simulink model "Heli_Server"  (Simulink 7.6)
settings: Solver=ode4  SolverMode=SingleTasking  StartTime=0.0  StopTime=inf  FixedStep=0.001  MaxStep=1e-2  RelTol=1e-3
values from neighbouring files (symbols this model uses):
  D = 0.9    [exp_doc.mat]
undefined symbols (not defined in the file or in its folder): A_dlon_nom, a_mr, a_tr, B_dlat_nom, C_D0_mr, C_D0_tr, C_La_ht, C_La_vf, eps_vf_tr, g_f, g_i, gamma_fb, h_mr, h_tr, I_rot, I_xx, I_yy, I_zz, K_beta, K_i, K_mu, K_p, l_ht, l_tr, m, n_tr, Omega_nom, R_mr, R_tr, rho, s, S_ht, S_vf, S_x_fus, S_y_fus, S_z_fus, sigma_mr, sigma_tr, x0_mod
libraries: aerolib6dofsys x3, aerolibconvert2 x2, simulink x2, aerolibutil x1
settings Model: Creator=jordan  LastModifiedBy=jordan
settings DataIOCC: LimitDataPoints=off  SaveOutput=off  SignalLogging=off  DSMLogging=off  SaveTime=off
settings OptimizationCC: OptimizeModelRefInitCode=on  LifeSpan=Inf
settings HardwareCC: ProdIntDivRoundTo=Zero  ProdEndianess=LittleEndian  ProdHWDeviceType=Generic->32-bit x86 compatible
settings RTWCC: SystemTargetFile=ert.tlc  TemplateMakefile=RTW.MSVCBuild  Description=Create Visual C/C++ Solution File for the Real-Time Workshop Embedded Coder  ProcessScript=ert_make_rtw_hook  RTWCompilerOptimization=On
settings CodeAppCC: IgnoreCustomStorageClasses=off  MaxIdLength=95
settings ERTTargetCC: MultiwordLength=2048  GenerateSampleERTMain=on  LogVarNameModifier=none  MatFileLogging=on  SupportContinuousTime=on  SupportNonInlinedSFcns=on  ERTCustomFileTemplate=example_file_process.tlc  ConvertIfToSwitch=off

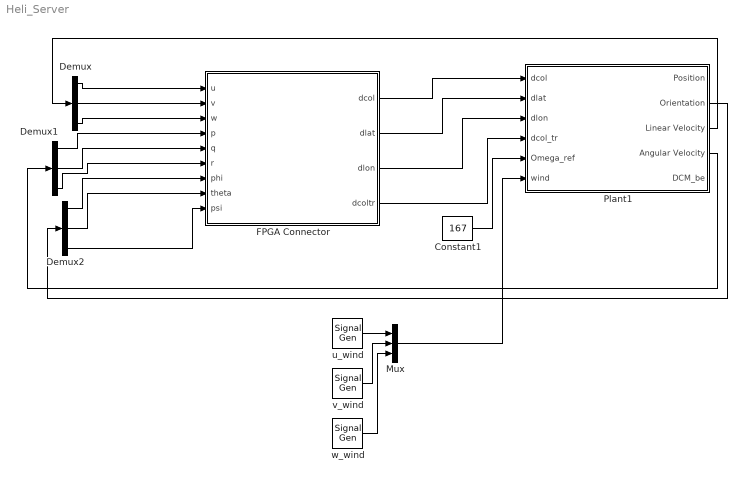
== system Heli_Server ==
  Constant1 : Constant  Value=167
  Demux : Demux  Outputs=3
  Demux1 : Demux  Outputs=3
  Demux2 : Demux  Outputs=3
  FPGA Connector : Subsystem
  Mux : Mux  Inputs=3
  Plant1 : Subsystem
  u_wind : SignalGenerator  WaveForm=square  Amplitude=5  Frequency=0.05
  v_wind : SignalGenerator  WaveForm=square  Amplitude=0.0  Frequency=0.04
  w_wind : SignalGenerator  WaveForm=square  Amplitude=0.0  Frequency=0.02
  wires:
  Plant1/3(Linear Velocity) -> Demux/1
  Plant1/4(Angular Velocity) -> Demux1/1
  Demux/1 -> FPGA Connector/1(u)
  Demux/2 -> FPGA Connector/2(v)
  Demux/3 -> FPGA Connector/3(w)
  Demux1/1 -> FPGA Connector/4(p)
  Demux1/2 -> FPGA Connector/5(q)
  Demux1/3 -> FPGA Connector/6(r)
  Demux2/1 -> FPGA Connector/7(phi)
  Demux2/2 -> FPGA Connector/8(theta)
  Demux2/3 -> FPGA Connector/9(psi)
  FPGA Connector/1(dcol) -> Plant1/1(dcol)
  FPGA Connector/4(dcoltr) -> Plant1/4(dcol_tr)
  Constant1/1 -> Plant1/5(Omega_ref)
  Plant1/2(Orientation) -> Demux2/1
  FPGA Connector/2(dlat) -> Plant1/2(dlat)
  FPGA Connector/3(dlon) -> Plant1/3(dlon)
  Mux/1 -> Plant1/6(wind)
  u_wind/1 -> Mux/1
  v_wind/1 -> Mux/2
  w_wind/1 -> Mux/3

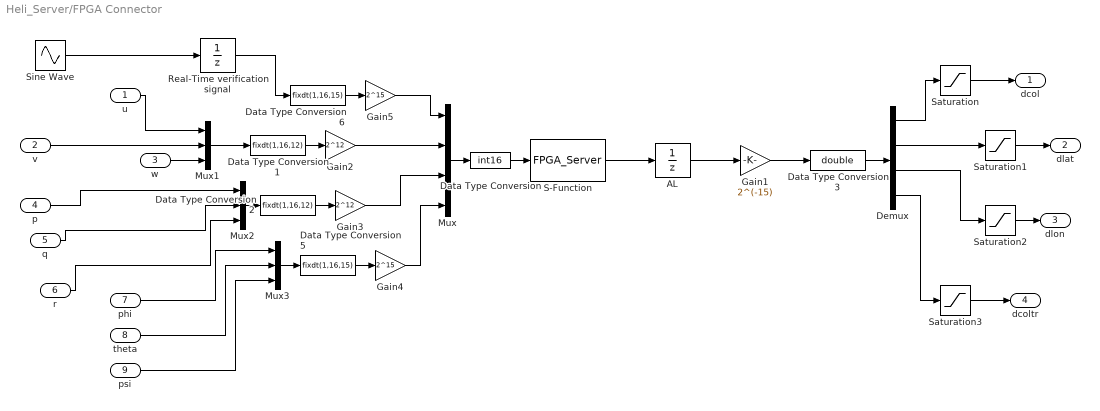
== system Heli_Server/FPGA Connector ==
  u : Inport
  v : Inport  Port=2
  w : Inport  Port=3
  p : Inport  Port=4
  q : Inport  Port=5
  r : Inport  Port=6
  phi : Inport  Port=7
  theta : Inport  Port=8
  psi : Inport  Port=9
  AL : UnitDelay  SampleTime=0.001
  Data Type Conversion : DataTypeConversion  OutDataTypeStr=int16  SaturateOnIntegerOverflow=on
  Data Type Conversion1 : DataTypeConversion  OutDataTypeStr=fixdt(1,16,12)  SaturateOnIntegerOverflow=on
  Data Type Conversion2 : DataTypeConversion  OutDataTypeStr=fixdt(1,16,12)  SaturateOnIntegerOverflow=on
  Data Type Conversion3 : DataTypeConversion  OutDataTypeStr=double  SaturateOnIntegerOverflow=on
  Data Type Conversion5 : DataTypeConversion  OutDataTypeStr=fixdt(1,16,15)  SaturateOnIntegerOverflow=on
  Data Type Conversion6 : DataTypeConversion  OutDataTypeStr=fixdt(1,16,15)  SaturateOnIntegerOverflow=on
  Demux : Demux
  Gain1 : Gain  Gain=2^(-15)  OutDataTypeStr=fixdt(1,16,15)
  Gain2 : Gain  Gain=2^12  OutDataTypeStr=int16
  Gain3 : Gain  Gain=2^12  OutDataTypeStr=int16
  Gain4 : Gain  Gain=2^15  OutDataTypeStr=int16
  Gain5 : Gain  Gain=2^15  OutDataTypeStr=int16
  Mux : Mux
  Mux1 : Mux  Inputs=3
  Mux2 : Mux  Inputs=3
  Mux3 : Mux  Inputs=3
  Real-Time verification signal : UnitDelay  SampleTime=0.001
  S-Function : S-Function  FunctionName=FPGA_Server  EnableBusSupport=off
  Saturation : Saturate  UpperLimit=0.183  LowerLimit=-0.183
  Saturation1 : Saturate  UpperLimit=0.096  LowerLimit=-0.096
  Saturation2 : Saturate  UpperLimit=0.096  LowerLimit=-0.096
  Saturation3 : Saturate  UpperLimit=0.48  LowerLimit=-0.48
  Sine Wave : Sin  Amplitude=0.3  Frequency=2*pi  SampleTime=0
  dcol : Outport
  dlat : Outport  Port=2
  dlon : Outport  Port=3
  dcoltr : Outport  Port=4
  wires:
  S-Function/1 -> AL/1
  Mux/1 -> Data Type Conversion/1
  Sine Wave/1 -> Real-Time verification signal/1
  Demux/1 -> Saturation/1
  Real-Time verification signal/1 -> Data Type Conversion6/1
  Data Type Conversion/1 -> S-Function/1
  Gain5/1 -> Mux/1
  u/1 -> Mux1/1
  v/1 -> Mux1/2
  p/1 -> Mux2/1
  q/1 -> Mux2/2
  r/1 -> Mux2/3
  phi/1 -> Mux3/1
  theta/1 -> Mux3/2
  psi/1 -> Mux3/3
  Demux/2 -> Saturation1/1
  Demux/3 -> Saturation2/1
  Demux/4 -> Saturation3/1
  Gain1/1 -> Data Type Conversion3/1
  AL/1 -> Gain1/1
  Data Type Conversion3/1 -> Demux/1
  Mux1/1 -> Data Type Conversion1/1
  Gain2/1 -> Mux/2
  Data Type Conversion2/1 -> Gain3/1
  Mux2/1 -> Data Type Conversion2/1
  Gain3/1 -> Mux/3
  Data Type Conversion5/1 -> Gain4/1
  Mux3/1 -> Data Type Conversion5/1
  Gain4/1 -> Mux/4
  Data Type Conversion6/1 -> Gain5/1
  Saturation/1 -> dcol/1
  Saturation1/1 -> dlat/1
  Saturation2/1 -> dlon/1
  Saturation3/1 -> dcoltr/1
  w/1 -> Mux1/3
  Data Type Conversion1/1 -> Gain2/1

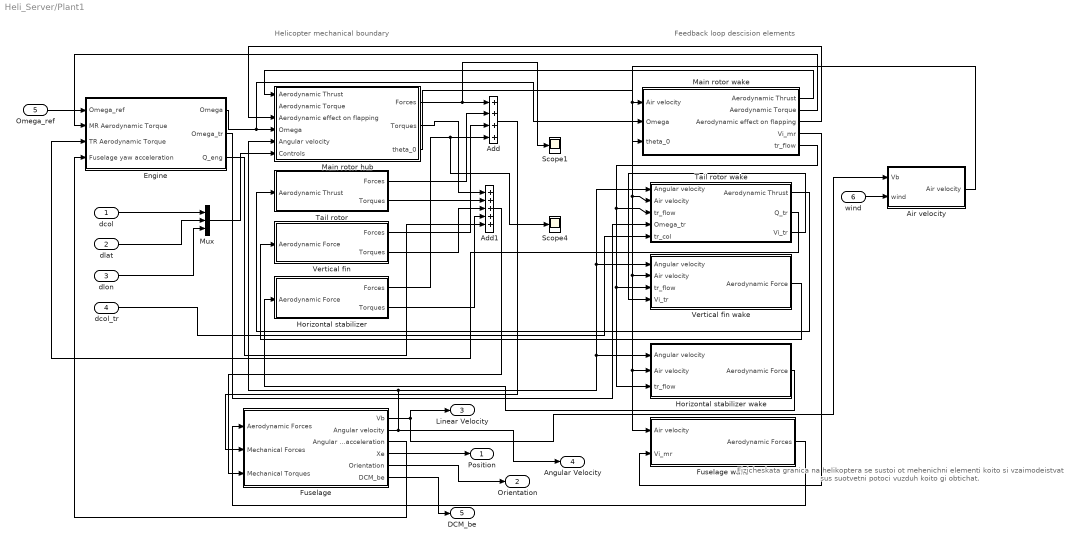
== system Heli_Server/Plant1 ==
  note: Fizicheskata granica na helikoptera
      | se sustoi ot mehenichni elementi
      | koito si vzaimodeistvat sus suotvetni
      | potoci vuzduh koito gi obtichat.
  note: Feedback loop descision elements
  note: Helicopter mechanical boundary
  dcol : Inport
  dlat : Inport  Port=2
  dlon : Inport  Port=3
  dcol_tr : Inport  Port=4
  Omega_ref : Inport  Port=5
  wind : Inport  Port=6
  Add : Sum  Inputs=++++
  Add1 : Sum  Inputs=+++++
  Air velocity : Subsystem
  Engine : Subsystem
  Fuselage : Subsystem
  Fuselage wake : Subsystem
  Horizontal stabilizer : Subsystem
  Horizontal stabilizer wake : Subsystem
  Main rotor hub : Subsystem
  Main rotor wake : Subsystem
  Mux : Mux  Inputs=3
  Scope1 : Scope
      settings: SaveName=ScopeData30
  Scope4 : Scope
      settings: SaveName=ScopeData34
  Tail rotor : Subsystem
  Tail rotor wake : Subsystem
  Vertical fin : Subsystem
  Vertical fin wake : Subsystem
  Position : Outport
  Orientation : Outport  Port=2
  Linear Velocity : Outport  Port=3
  Angular Velocity : Outport  Port=4
  DCM_be : Outport  Port=5
  wires:
  Vertical fin/1(Forces) -> Add/3
  Engine/3(Q_eng) -> Add1/5
  Tail rotor wake/2(Q_tr) -> Engine/3(TR Aerodynamic Torque)
  Fuselage/6(DCM_be) -> DCM_be/1
  wind/1 -> Air velocity/2(wind)
  Omega_ref/1 -> Engine/1(Omega_ref)
  Fuselage/5(Orientation) -> Orientation/1
  Fuselage/4(Xe) -> Position/1
  dcol_tr/1 -> Tail rotor wake/5(tr_col)
  dlon/1 -> Mux/3
  dlat/1 -> Mux/2
  dcol/1 -> Mux/1
  Horizontal stabilizer/2(Torques) -> Add1/4
  Vertical fin/2(Torques) -> Add1/3
  Tail rotor/2(Torques) -> Add1/2
  Main rotor hub/2(Torques) -> Add1/1
  Add1/1 -> Fuselage/3(Mechanical Torques)
  Horizontal stabilizer/1(Forces) -> Scope4/1, Add/4
  Tail rotor/1(Forces) -> Add/2
  Add/1 -> Fuselage/2(Mechanical Forces)
  Horizontal stabilizer wake/1(Aerodynamic Force) -> Horizontal stabilizer/1(Aerodynamic Force)
  Vertical fin wake/1(Aerodynamic Force) -> Vertical fin/1(Aerodynamic Force)
  Tail rotor wake/1(Aerodynamic Thrust) -> Tail rotor/1(Aerodynamic Thrust)
  Engine/2(Omega_tr) -> Tail rotor wake/4(Omega_tr)
  Main rotor wake/5(tr_flow) -> Tail rotor wake/3(tr_flow), Horizontal stabilizer wake/3(tr_flow), Vertical fin wake/3(tr_flow)
  Mux/1 -> Main rotor hub/6(Controls)
  Main rotor hub/1(Forces) -> Scope1/1, Add/1
  Main rotor hub/3(theta_0) -> Main rotor wake/3(theta_0)
  Main rotor wake/3(Aerodynamic effect on flapping) -> Main rotor hub/3(Aerodynamic effect on flapping)
  Fuselage/3(Angular acceleration) -> Engine/4(Fuselage yaw acceleration)
  Tail rotor wake/3(Vi_tr) -> Vertical fin wake/4(Vi_tr)
  Fuselage/2(Angular velocity) -> Angular Velocity/1, Horizontal stabilizer wake/1(Angular velocity), Tail rotor wake/1(Angular velocity), Vertical fin wake/1(Angular velocity), Main rotor hub/5(Angular velocity)
  Fuselage wake/1(Aerodynamic Forces) -> Fuselage/1(Aerodynamic Forces)
  Main rotor wake/4(Vi_mr) -> Fuselage wake/2(Vi_mr)
  Main rotor wake/2(Aerodynamic Torque) -> Engine/2(MR Aerodynamic Torque)
  Air velocity/1(Air velocity) -> Main rotor wake/1(Air velocity), Tail rotor wake/2(Air velocity), Horizontal stabilizer wake/2(Air velocity), Fuselage wake/1(Air velocity), Vertical fin wake/2(Air velocity)
  Fuselage/1(Vb) -> Linear Velocity/1, Air velocity/1(Vb)
  Main rotor wake/1(Aerodynamic Thrust) -> Main rotor hub/1(Aerodynamic Thrust)
  Engine/1(Omega) -> Main rotor wake/2(Omega), Main rotor hub/4(Omega)

== system Heli_Server/Plant1/Air velocity ==
  Vb : Inport
  wind : Inport  Port=2
  Add : Sum  Inputs=-+
  Air velocity : Outport
  wires:
  Add/1 -> Air velocity/1
  Vb/1 -> Add/2
  wind/1 -> Add/1

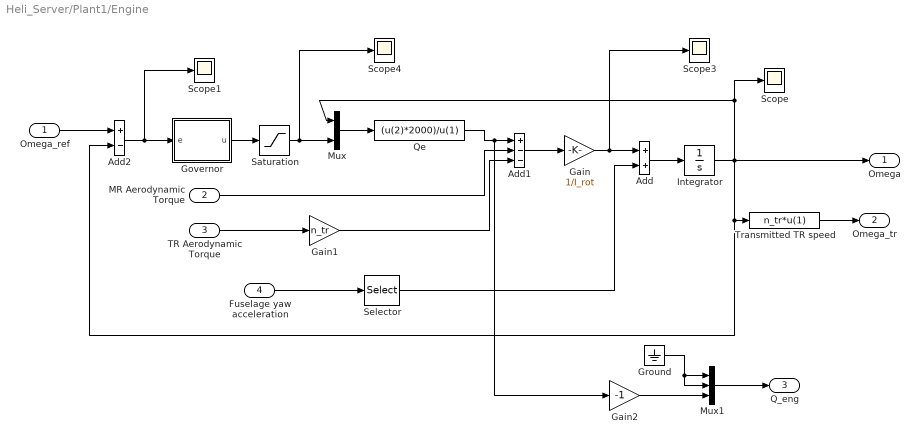
== system Heli_Server/Plant1/Engine ==
  Omega_ref : Inport
  MR Aerodynamic Torque : Inport  Port=2
  TR Aerodynamic Torque : Inport  Port=3
  Fuselage yaw acceleration : Inport  Port=4
  Add : Sum
  Add1 : Sum  Inputs=+--
  Add2 : Sum  Inputs=+-
  Gain : Gain  Gain=1/I_rot
  Gain1 : Gain  Gain=n_tr
  Gain2 : Gain  Gain=-1
  Governor : Subsystem
  Ground : Ground
  Integrator : Integrator  InitialCondition=167  UpperSaturationLimit=200  LowerSaturationLimit=150  ContinuousStateAttributes='Omega'
  Mux : Mux  Inputs=2
  Mux1 : Mux  Inputs=3
  Qe : Fcn  Expr=(u(2)*2000)/u(1)
  Saturation : Saturate  UpperLimit=1  LowerLimit=-1
  Scope{,1,3..4} (4 alike) : Scope
      Scope settings: TimeRange=10  YMin=166  YMax=168.5  SaveName=ScopeData28
      Scope1 settings: TimeRange=10  YMin=-1.5  YMax=0.25  SaveName=ScopeData31
      Scope3 settings: TimeRange=10  YMin=166  YMax=168.5  SaveName=ScopeData26
      Scope4 settings: TimeRange=10  YMin=-1.5  YMax=0.25  SaveName=ScopeData27
  Selector : Selector  InputPortWidth=3  IndexOptions=Index vector (dialog)  Indices=3  OutputSizes=1
  Transmitted TR speed : Fcn  Expr=n_tr*u(1)
  Omega : Outport
  Omega_tr : Outport  Port=2
  Q_eng : Outport  Port=3
  wires:
  Mux1/1 -> Q_eng/1
  Ground/1 -> Mux1/2, Mux1/1
  Gain2/1 -> Mux1/3
  Gain1/1 -> Add1/3
  Mux/1 -> Qe/1
  Qe/1 -> Gain2/1, Add1/1
  Saturation/1 -> Scope4/1, Mux/2
  Governor/1(u) -> Saturation/1
  Add2/1 -> Governor/1(e), Scope1/1
  Omega_ref/1 -> Add2/1
  TR Aerodynamic Torque/1 -> Gain1/1
  MR Aerodynamic Torque/1 -> Add1/2
  Gain/1 -> Scope3/1, Add/1
  Add1/1 -> Gain/1
  Selector/1 -> Add/2
  Add/1 -> Integrator/1
  Fuselage yaw acceleration/1 -> Selector/1
  Transmitted TR speed/1 -> Omega_tr/1
  Integrator/1 -> Omega/1, Mux/1, Scope/1, Add2/2, Transmitted TR speed/1

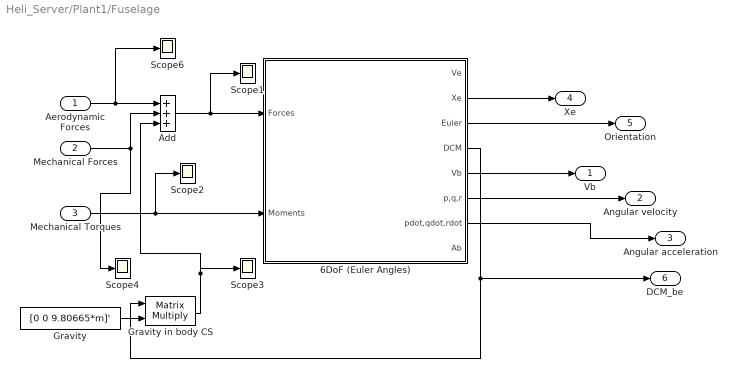
== system Heli_Server/Plant1/Fuselage ==
  Aerodynamic Forces : Inport
  Mechanical Forces : Inport  Port=2
  Mechanical Torques : Inport  Port=3
  6DoF (Euler Angles) : Subsystem  AncestorBlock=aerolib6dof2/6DoF (Euler Angles)  mask(6DoF EoM (Body Axis)){units=Metric (MKS), mtype=Fixed, rep=Euler Angles, xme_0=[0 0 0], Vm_0=[0 0 0], eul_0=[0 0 0], pm_0=[0 0 0], mass_0=m, mass_e=0.5, mass_f=2.0, inertia=[I_xx 0 0;0 I_yy 0;0 0 I_zz], inertia_e=eye(3), inertia_f=2*eye(3), k_quat=1.0}
      mask prompts: mtype "Mass type:"; rep "Representation:"; xme_0 "Initial position in inertial axes [Xe,Ye,Ze]:"; Vm_0 "Initial velocity in body axes [U,v,w]:"; eul_0 "Initial Euler orientation [roll, pitch, yaw]:"; pm_0 "Initial body rotation rates [p,q,r]:"; mass_0 "Initial mass:"; mass_e "Empty mass:"; mass_f "Full mass:"; inertia_e "Empty inertia matrix:"; inertia_f "Full inertia matrix:"; k_quat "Gain for quaternion normalization:"
      mask help: Integrate the six-degrees-of-freedom equations of motion in body axis.
      mask init:
      | [x y xp yp highstr lowstr maxy miny]=aeroimage('sixdofbody',gcbh);
      | ports=aeroicon('aeroblk6dofbody','icon');
      mask Help: eval('asbhelp(''sixdof_euler_angles'')');
      mask StyleString: popup(Metric (MKS)|English (Velocity in ft/s)|English (Velocity in kts)),popup(Fixed|Simple Variable|Custom Variable),popup(Euler Angles|Quaternion),edit,edit,edit,edit,edit,edit,edit,edit,edit,edit,edit
      mask CallbackString: |aeroicon('aeroblk6dofbody');|aeroicon('aeroblk6dofbody');|||||||||||
      mask Display:
      | port_label(ports(1).type,ports(1).port,ports(1).txt,'texmode','on');
      | port_label(ports(2).type,ports(2).port,ports(2).txt,'texmode','on');
      | port_label(ports(3).type,ports(3).port,ports(3).txt,'texmode','on');
      | port_label(ports(4).type,ports(4).port,ports(4).txt,'texmode','on');
      | port_label(ports(5).type,ports(5).port,ports(5).txt,'texmode','on');
      | port_label(ports(6).type,ports(6).port,ports(6).txt,'texmode','on');
      | port_label(ports(7).type,ports(7).port,ports(7).txt,'texmode','on');
      | port_label(ports(8).type,ports(8).port,ports(8).txt,'texmode','on');
      | port_label(ports(9).type,ports(9).port,ports(9).txt,'texmode','on');
      | port_label(ports(10).type,ports(10).port,ports(10).txt,'texmode','on');
      | port_label(ports(11).type,ports(11).port,ports(11).txt,'texmode','on');
      | port_label(ports(12).type,ports(12).port,ports(12).txt,'texmode','on');
      | port_label(ports(13).type,ports(13).port,ports(13).txt,'texmode','on');
      | port_label(ports(14).type,ports(14).port,ports(14).txt,'texmode','on');
      | port_label(ports(15).type,ports(15).port,ports(15).txt,'texmode','on');
      | text(0.5,maxy+0.065,highstr{:},'horizontalAlignment','center')
      | text(0.5,miny-0.05,lowstr{:},'horizontalAlignment','center')
      | plot(x,y);
      | patch(xp, yp);
  Add : Sum  Inputs=+++
  Gravity : Constant  Value=[0 0 9.80665*m]'
  Gravity in body CS : Product  Multiplication=Matrix(*)  RndMeth=Zero
  Scope{1..4,6} (5 alike) : Scope
      Scope3 settings: SaveName=ScopeData19
      Scope4 settings: SaveName=ScopeData29
      Scope6 settings: SaveName=ScopeData23
  Vb : Outport
  Angular velocity : Outport  Port=2
  Angular acceleration : Outport  Port=3
  Xe : Outport  Port=4
  Orientation : Outport  Port=5
  DCM_be : Outport  Port=6
  wires:
  6DoF (Euler Angles)/3(Euler) -> Orientation/1
  6DoF (Euler Angles)/2(Xe) -> Xe/1
  Gravity in body CS/1 -> Scope3/1, Add/3
  Gravity/1 -> Gravity in body CS/2
  6DoF (Euler Angles)/4(DCM) -> DCM_be/1, Gravity in body CS/1
  6DoF (Euler Angles)/5(Vb) -> Vb/1
  6DoF (Euler Angles)/7(pdot,qdot,rdot) -> Angular acceleration/1
  6DoF (Euler Angles)/6(p,q,r) -> Angular velocity/1
  Mechanical Torques/1 -> 6DoF (Euler Angles)/2(Moments), Scope2/1
  Add/1 -> 6DoF (Euler Angles)/1(Forces), Scope1/1
  Mechanical Forces/1 -> Scope4/1, Add/2
  Aerodynamic Forces/1 -> Add/1, Scope6/1

== system Heli_Server/Plant1/Fuselage wake ==
  Air velocity : Inport
  Vi_mr : Inport  Port=2
  Mux : Mux  Inputs=2
  Mux1 : Mux  Inputs=3
  Mux2 : Mux  Inputs=2
  V_inf : Fcn  Expr=sqrt(u(1)^2+u(2)^2+(u(3)+u(4))^2)
  X_fus : Fcn  Expr=-0.5*rho*S_x_fus*u(1)*u(5)
  Y_fus : Fcn  Expr=-0.5*rho*S_y_fus*u(2)*u(5)
  Z_fus : Fcn  Expr=-0.5*rho*S_z_fus*(u(3)+u(4))*u(5)
  Aerodynamic Forces : Outport
  wires:
  Z_fus/1 -> Mux1/3
  Y_fus/1 -> Mux1/2
  X_fus/1 -> Mux1/1
  Mux2/1 -> Z_fus/1, Y_fus/1, X_fus/1
  V_inf/1 -> Mux2/2
  Mux1/1 -> Aerodynamic Forces/1
  Mux/1 -> Mux2/1, V_inf/1
  Vi_mr/1 -> Mux/2
  Air velocity/1 -> Mux/1

== system Heli_Server/Plant1/Horizontal stabilizer ==
  Aerodynamic Force : Inport
  Ground : Ground
  Mux : Mux  Inputs=3
  Mux1 : Mux  Inputs=3
  pitch torque : Fcn  Expr=u(1)*l_ht
  Forces : Outport
  Torques : Outport  Port=2
  wires:
  pitch torque/1 -> Mux1/2
  Mux/1 -> Forces/1
  Aerodynamic Force/1 -> Mux/3, pitch torque/1
  Ground/1 -> Mux/2, Mux1/1, Mux1/3, Mux/1
  Mux1/1 -> Torques/1

== system Heli_Server/Plant1/Horizontal stabilizer wake ==
  Angular velocity : Inport
  Air velocity : Inport  Port=2
  tr_flow : Inport  Port=3
  Gain : Gain  Gain=-1
  Mux : Mux  Inputs=3
  Mux2 : Mux  Inputs=2
  Z_ht : simulink/Discontinuities/Saturation Dynamic  SystemSampleTime=-1  OutMin=[]  OutMax=[]  OutDataTypeStr=Inherit: Same as second input  OutDataType=fixdt(1, 16)  OutScaling=2^-10  DoSatur=off
  Z_ht_ideal : Fcn  Expr=0.5*rho*S_ht*(C_La_ht*abs(u(1))*u(4)+abs(u(4))*u(4))
  Z_ht_max : Fcn  Expr=0.5*rho*S_ht*(u(1)^2+u(4)^2)
  w_ht : Fcn  Expr=u(6)+l_ht*u(2)-u(7)
  Aerodynamic Force : Outport
  wires:
  Z_ht/1 -> Aerodynamic Force/1
  Gain/1 -> Z_ht/3
  Z_ht_max/1 -> Gain/1, Z_ht/1
  Z_ht_ideal/1 -> Z_ht/2
  Mux2/1 -> Z_ht_max/1, Z_ht_ideal/1
  w_ht/1 -> Mux2/2
  tr_flow/1 -> Mux/3
  Air velocity/1 -> Mux2/1, Mux/2
  Angular velocity/1 -> Mux/1
  Mux/1 -> w_ht/1

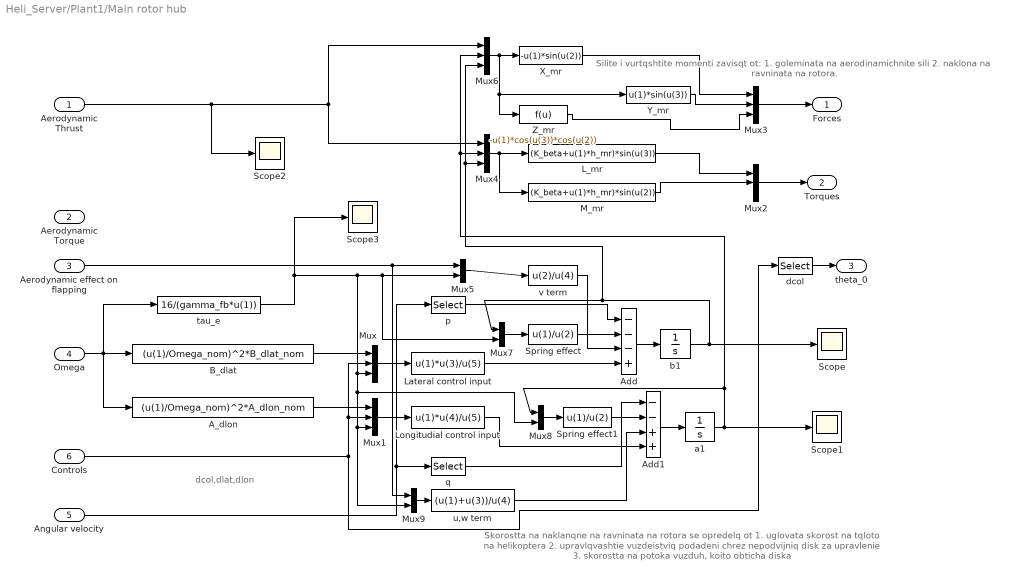
== system Heli_Server/Plant1/Main rotor hub ==
  note: dcol,dlat,dlon
  note: Skorostta na naklanqne na ravninata na rotora se opredelq ot
      | 1. uglovata skorost na tqloto na helikoptera
      | 2. upravlqvashtie vuzdeistviq podadeni chrez
      | nepodvijniq disk za upravlenie
      | 3. skorostta na potoka vuzduh, koito obticha diska
  note: Silite i vurtqshtite momenti zavisqt ot:
      | 1. goleminata na aerodinamichnite sili
      | 2. naklona na ravninata na rotora.
  Aerodynamic Thrust : Inport
  Aerodynamic Torque : Inport  Port=2
  Aerodynamic effect on flapping : Inport  Port=3
  Omega : Inport  Port=4
  Angular velocity : Inport  Port=5
  Controls : Inport  Port=6
  A_dlon : Fcn  Expr=(u(1)/Omega_nom)^2*A_dlon_nom
  Add : Sum  Inputs=---+
  Add1 : Sum  Inputs=--++
  B_dlat : Fcn  Expr=(u(1)/Omega_nom)^2*B_dlat_nom
  L_mr : Fcn  Expr=(K_beta+u(1)*h_mr)*sin(u(3))
  Lateral control input : Fcn  Expr=u(1)*u(3)/u(5)
  Longitudial control input : Fcn  Expr=u(1)*u(4)/u(5)
  M_mr : Fcn  Expr=(K_beta+u(1)*h_mr)*sin(u(2))
  Mux{,1..4,6} (6 alike) : Mux  Inputs=3
  Mux{5,7..9} (4 alike) : Mux  Inputs=2
  Scope{,1..3} (4 alike) : Scope
      Scope settings: SaveName=ScopeData2
      Scope1 settings: SaveName=ScopeData3
      Scope2 settings: SaveName=ScopeData35
      Scope3 settings: SaveName=ScopeData18
  Spring effect : Fcn  Expr=u(1)/u(2)
  Spring effect1 : Fcn  Expr=u(1)/u(2)
  X_mr : Fcn  Expr=-u(1)*sin(u(2))
  Y_mr : Fcn  Expr=u(1)*sin(u(3))
  Z_mr : Fcn  Expr=-u(1)*cos(u(3))*cos(u(2))
  a1 : Integrator  InitialCondition=x0_mod(12)
  b1 : Integrator  InitialCondition=x0_mod(13)
  dcol : Selector  InputPortWidth=3  IndexOptions=Index vector (dialog)  Indices=1  OutputSizes=1
  p : Selector  InputPortWidth=3  IndexOptions=Index vector (dialog)  Indices=1  OutputSizes=1
  q : Selector  InputPortWidth=3  IndexOptions=Index vector (dialog)  Indices=2  OutputSizes=1
  tau_e : Fcn  Expr=16/(gamma_fb*u(1))
  u,w term : Fcn  Expr=(u(1)+u(3))/u(4)
  v term : Fcn  Expr=u(2)/u(4)
  Forces : Outport
  Torques : Outport  Port=2
  theta_0 : Outport  Port=3
  wires:
  Mux9/1 -> u,w term/1
  Mux8/1 -> Spring effect1/1
  Mux7/1 -> Spring effect/1
  tau_e/1 -> Scope3/1, Mux9/2, Mux1/3, Mux8/2, Mux/3, Mux7/2, Mux5/2
  Mux5/1 -> v term/1
  Aerodynamic effect on flapping/1 -> Mux9/1, Mux5/1
  dcol/1 -> theta_0/1
  Z_mr/1 -> Mux3/3
  Y_mr/1 -> Mux3/2
  X_mr/1 -> Mux3/1
  Mux6/1 -> Z_mr/1, Y_mr/1, X_mr/1
  M_mr/1 -> Mux2/2
  L_mr/1 -> Mux2/1
  Aerodynamic Thrust/1 -> Scope2/1, Mux6/1, Mux4/1
  Mux4/1 -> M_mr/1, L_mr/1
  Mux3/1 -> Forces/1
  Mux2/1 -> Torques/1
  Longitudial control input/1 -> Add1/4
  Spring effect1/1 -> Add1/2
  Add1/1 -> a1/1
  u,w term/1 -> Add1/3
  a1/1 -> Scope1/1, Mux8/1, Mux4/2, Mux6/2
  q/1 -> Add1/1
  Angular velocity/1 -> q/1, p/1
  v term/1 -> Add/3
  Spring effect/1 -> Add/2
  b1/1 -> Scope/1, Mux7/1, Mux4/3, Mux6/3
  Add/1 -> b1/1
  Lateral control input/1 -> Add/4
  p/1 -> Add/1
  Mux1/1 -> Longitudial control input/1
  A_dlon/1 -> Mux1/1
  Mux/1 -> Lateral control input/1
  Controls/1 -> dcol/1, Mux/2, Mux1/2
  B_dlat/1 -> Mux/1
  Omega/1 -> tau_e/1, A_dlon/1, B_dlat/1

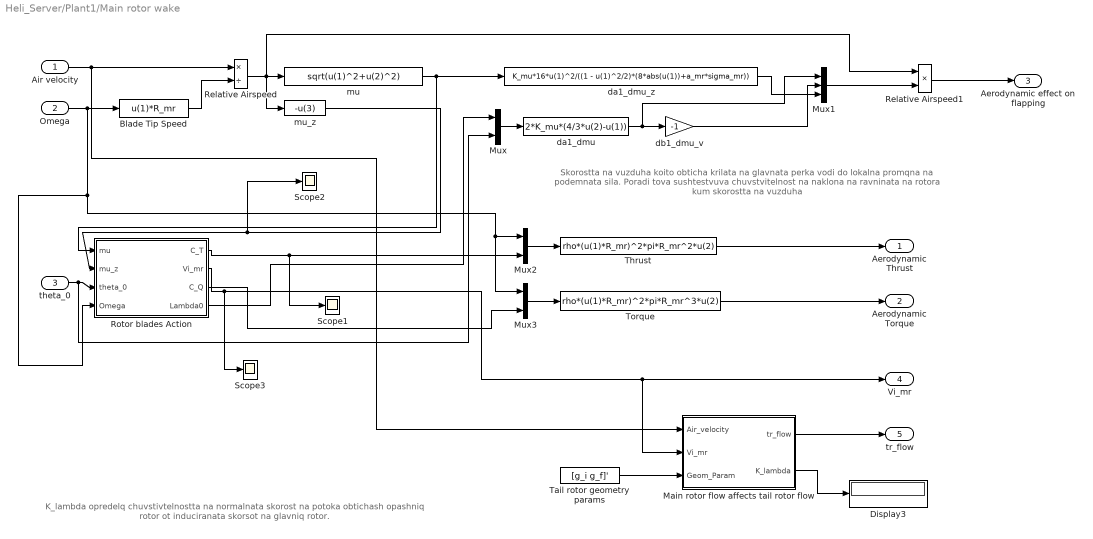
== system Heli_Server/Plant1/Main rotor wake ==
  note: Skorostta na vuzduha koito obticha krilata na glavnata
      | perka vodi do lokalna promqna na podemnata sila.
      | Poradi tova sushtestvuva chuvstvitelnost na naklona
      | na ravninata na rotora kum skorostta na vuzduha
  note: K_lambda opredelq chuvstivtelnostta na
      | normalnata skorost na potoka obtichash
      | opashniq rotor ot induciranata skorsot na
      | glavniq rotor.
  Air velocity : Inport  PortDimensions=3
  Omega : Inport  Port=2
  theta_0 : Inport  Port=3
  Blade Tip Speed : Fcn  Expr=u(1)*R_mr
  Display3 : Display
  Main rotor flow affects tail rotor flow : Stateflow chart  TreatAsAtomicUnit=on
  Mux : Mux  Inputs=2
  Mux1 : Mux  Inputs=3
  Mux2 : Mux  Inputs=2
  Mux3 : Mux  Inputs=2
  Relative Airspeed : Product  Inputs=*/
  Relative Airspeed1 : Product  Inputs=**
  Rotor blades Action : Subsystem
  Scope1 : Scope
      settings: SaveName=ScopeData11
  Scope2 : Scope
      settings: SaveName=ScopeData10
  Scope3 : Scope
      settings: SaveName=ScopeData12
  Tail rotor geometry params : Constant  Value=[g_i g_f]'
  Thrust : Fcn  Expr=rho*(u(1)*R_mr)^2*pi*R_mr^2*u(2)
  Torque : Fcn  Expr=rho*(u(1)*R_mr)^2*pi*R_mr^3*u(2)
  da1_dmu : Fcn  Expr=2*K_mu*(4/3*u(2)-u(1))
  da1_dmu_z : Fcn  Expr=K_mu*16*u(1)^2/((1 - u(1)^2/2)*(8*abs(u(1))+a_mr*sigma_mr))
  db1_dmu_v : Gain  Gain=-1
  mu : Fcn  Expr=sqrt(u(1)^2+u(2)^2)
  mu_z : Fcn  Expr=-u(3)
  Aerodynamic Thrust : Outport
  Aerodynamic Torque : Outport  Port=2
  Aerodynamic effect on flapping : Outport  Port=3
  Vi_mr : Outport  Port=4
  tr_flow : Outport  Port=5
  wires:
  Main rotor flow affects tail rotor flow/2(K_lambda) -> Display3/1
  Mux3/1 -> Torque/1
  Torque/1 -> Aerodynamic Torque/1
  Air velocity/1 -> Relative Airspeed/1, Main rotor flow affects tail rotor flow/1(Air_velocity)
  Omega/1 -> Rotor blades Action/4(Omega), Mux3/1, Mux2/1, Blade Tip Speed/1
  Blade Tip Speed/1 -> Relative Airspeed/2
  Relative Airspeed/1 -> mu/1, mu_z/1, Relative Airspeed1/1
  mu/1 -> Rotor blades Action/1(mu), da1_dmu_z/1
  mu_z/1 -> Rotor blades Action/2(mu_z), Scope2/1
  theta_0/1 -> Rotor blades Action/3(theta_0), Mux/2
  Mux/1 -> da1_dmu/1
  Rotor blades Action/2(Vi_mr) -> Scope3/1, Vi_mr/1, Main rotor flow affects tail rotor flow/2(Vi_mr)
  da1_dmu/1 -> db1_dmu_v/1, Mux1/1
  da1_dmu_z/1 -> Mux1/3
  db1_dmu_v/1 -> Mux1/2
  Rotor blades Action/1(C_T) -> Mux2/2, Scope1/1
  Mux2/1 -> Thrust/1
  Thrust/1 -> Aerodynamic Thrust/1
  Rotor blades Action/3(C_Q) -> Mux3/2
  Main rotor flow affects tail rotor flow/1(tr_flow) -> tr_flow/1
  Tail rotor geometry params/1 -> Main rotor flow affects tail rotor flow/3(Geom_Param)
  Rotor blades Action/4(Lambda0) -> Mux/1
  Relative Airspeed1/1 -> Aerodynamic effect on flapping/1
  Mux1/1 -> Relative Airspeed1/2

== system Heli_Server/Plant1/Tail rotor ==
  note: Vurhu opashniqt rotor deistva tqgata
      | poluchena ot vurteneto na perkata.
      | Tova suzdava mehanichni sili vurhu tqloto
      | na helikoptera.
  Aerodynamic Thrust : Inport
  Ground : Ground
  Mux : Mux  Inputs=3
  Mux1 : Mux  Inputs=3
  roll torque : Fcn  Expr=u(1)*h_tr
  yaw torque : Fcn  Expr=-u(1)*l_tr
  Forces : Outport
  Torques : Outport  Port=2
  wires:
  roll torque/1 -> Mux1/1
  yaw torque/1 -> Mux1/3
  Mux1/1 -> Torques/1
  Ground/1 -> Mux1/2, Mux/3, Mux/1
  Aerodynamic Thrust/1 -> roll torque/1, yaw torque/1, Mux/2
  Mux/1 -> Forces/1

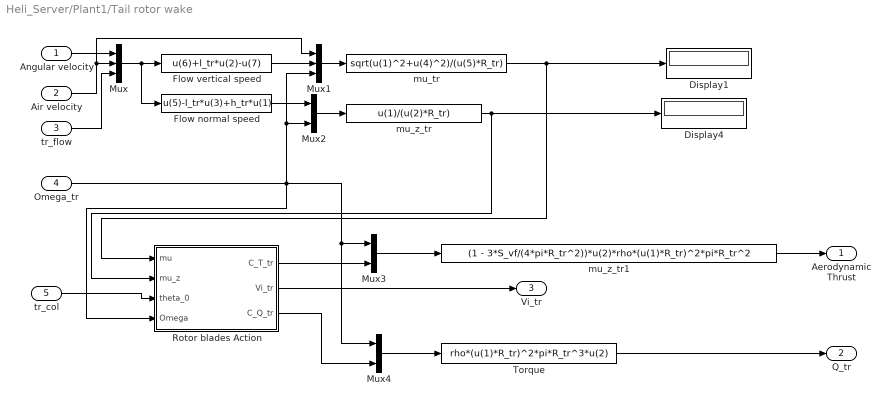
== system Heli_Server/Plant1/Tail rotor wake ==
  Angular velocity : Inport
  Air velocity : Inport  Port=2
  tr_flow : Inport  Port=3
  Omega_tr : Inport  Port=4
  tr_col : Inport  Port=5
  Display1 : Display
  Display4 : Display
  Flow normal speed : Fcn  Expr=u(5)-l_tr*u(3)+h_tr*u(1)
  Flow vertical speed : Fcn  Expr=u(6)+l_tr*u(2)-u(7)
  Mux : Mux  Inputs=3
  Mux1 : Mux  Inputs=3
  Mux2 : Mux  Inputs=2
  Mux3 : Mux  Inputs=2
  Mux4 : Mux  Inputs=2
  Rotor blades Action : Subsystem
  Torque : Fcn  Expr=rho*(u(1)*R_tr)^2*pi*R_tr^3*u(2)
  mu_tr : Fcn  Expr=sqrt(u(1)^2+u(4)^2)/(u(5)*R_tr)
  mu_z_tr : Fcn  Expr=u(1)/(u(2)*R_tr)
  mu_z_tr1 : Fcn  Expr=(1 - 3*S_vf/(4*pi*R_tr^2))*u(2)*rho*(u(1)*R_tr)^2*pi*R_tr^2
  Aerodynamic Thrust : Outport
  Q_tr : Outport  Port=2
  Vi_tr : Outport  Port=3
  wires:
  Air velocity/1 -> Mux/2, Mux1/1
  Angular velocity/1 -> Mux/1
  tr_flow/1 -> Mux/3
  Mux/1 -> Flow normal speed/1, Flow vertical speed/1
  Omega_tr/1 -> Rotor blades Action/4(Omega), Mux3/1, Mux4/1, Mux1/3, Mux2/2
  Mux1/1 -> mu_tr/1
  Mux2/1 -> mu_z_tr/1
  tr_col/1 -> Rotor blades Action/3(theta_0)
  mu_z_tr/1 -> Rotor blades Action/2(mu_z), Display4/1
  mu_z_tr1/1 -> Aerodynamic Thrust/1
  mu_tr/1 -> Rotor blades Action/1(mu), Display1/1
  Rotor blades Action/2(Vi_tr) -> Vi_tr/1
  Rotor blades Action/1(C_T_tr) -> Mux3/2
  Mux3/1 -> mu_z_tr1/1
  Torque/1 -> Q_tr/1
  Mux4/1 -> Torque/1
  Rotor blades Action/3(C_Q_tr) -> Mux4/2
  Flow vertical speed/1 -> Mux1/2
  Flow normal speed/1 -> Mux2/1

== system Heli_Server/Plant1/Vertical fin ==
  Aerodynamic Force : Inport
  Ground : Ground
  Mux : Mux  Inputs=3
  Mux1 : Mux  Inputs=3
  roll torque : Fcn  Expr=u(1)*h_tr
  yaw torque : Fcn  Expr=-u(1)*l_tr
  Forces : Outport
  Torques : Outport  Port=2
  wires:
  roll torque/1 -> Mux1/1
  yaw torque/1 -> Mux1/3
  Mux1/1 -> Torques/1
  Ground/1 -> Mux1/2, Mux/3, Mux/1
  Aerodynamic Force/1 -> roll torque/1, yaw torque/1, Mux/2
  Mux/1 -> Forces/1

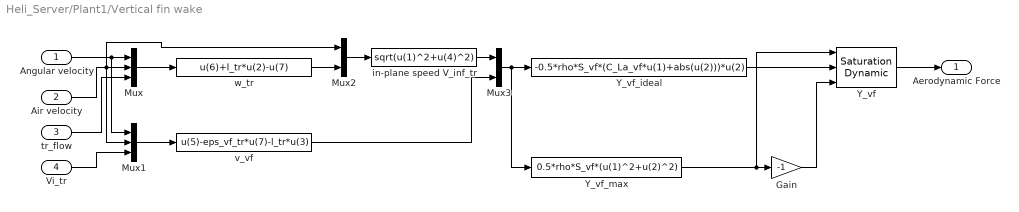
== system Heli_Server/Plant1/Vertical fin wake ==
  Angular velocity : Inport
  Air velocity : Inport  Port=2
  tr_flow : Inport  Port=3
  Vi_tr : Inport  Port=4
  Gain : Gain  Gain=-1
  Mux : Mux  Inputs=3
  Mux1 : Mux  Inputs=3
  Mux2 : Mux  Inputs=2
  Mux3 : Mux  Inputs=2
  Y_vf : simulink/Discontinuities/Saturation Dynamic  SystemSampleTime=-1  OutMin=[]  OutMax=[]  OutDataTypeStr=Inherit: Same as second input  OutDataType=fixdt(1, 16)  OutScaling=2^-10  DoSatur=off
  Y_vf_ideal : Fcn  Expr=-0.5*rho*S_vf*(C_La_vf*u(1)+abs(u(2)))*u(2)
  Y_vf_max : Fcn  Expr=0.5*rho*S_vf*(u(1)^2+u(2)^2)
  in-plane speed V_inf_tr : Fcn  Expr=sqrt(u(1)^2+u(4)^2)
  v_vf : Fcn  Expr=u(5)-eps_vf_tr*u(7)-l_tr*u(3)
  w_tr : Fcn  Expr=u(6)+l_tr*u(2)-u(7)
  Aerodynamic Force : Outport
  wires:
  Y_vf/1 -> Aerodynamic Force/1
  Gain/1 -> Y_vf/3
  Y_vf_max/1 -> Gain/1, Y_vf/1
  Y_vf_ideal/1 -> Y_vf/2
  Mux3/1 -> Y_vf_max/1, Y_vf_ideal/1
  v_vf/1 -> Mux3/2
  in-plane speed V_inf_tr/1 -> Mux3/1
  Mux2/1 -> in-plane speed V_inf_tr/1
  w_tr/1 -> Mux2/2
  Mux1/1 -> v_vf/1
  Vi_tr/1 -> Mux1/3
  tr_flow/1 -> Mux/3
  Air velocity/1 -> Mux2/1, Mux1/2, Mux/2
  Angular velocity/1 -> Mux1/1, Mux/1
  Mux/1 -> w_tr/1

== system Heli_Server/Plant1/Engine/Governor ==
  e : Inport
  Add3 : Sum
  Gain3 : Gain  Gain=K_p
  Gain4 : Gain  Gain=K_i
  Integrator1 : Integrator  InitialCondition=x0_mod(11)  UpperSaturationLimit=200  LowerSaturationLimit=150  ContinuousStateAttributes='Omega'
  Scope1 : Scope
      settings: TimeRange=10  YMin=-1.5  YMax=0.25  SaveName=ScopeData15
  u : Outport
  wires:
  Gain4/1 -> Scope1/1, Add3/2
  Add3/1 -> u/1
  e/1 -> Integrator1/1, Gain3/1
  Integrator1/1 -> Gain4/1
  Gain3/1 -> Add3/1

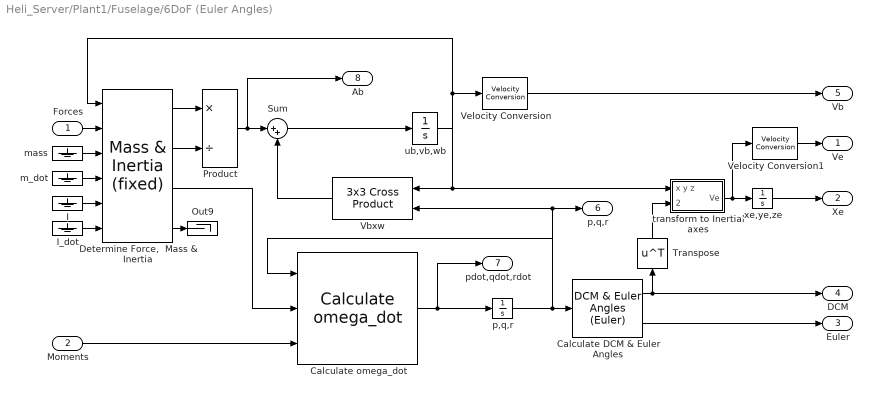
== system Heli_Server/Plant1/Fuselage/6DoF (Euler Angles) ==
  Forces : Inport
  Moments : Inport  Port=2
  Calculate DCM & Euler Angles : aerolib6dofsys/DCM & Euler Angles (Euler)  SystemSampleTime=-1
  Calculate omega_dot : aerolib6dofsys/Calculate omega_dot  SystemSampleTime=-1
  "Determine Force,  Mass & Inertia" : aerolib6dofsys/Mass & Inertia (fixed)  SystemSampleTime=-1
  I : Ground
  I_dot : Ground
  Out9 : Terminator
  Product : Product  Inputs=*/  SaturateOnIntegerOverflow=on  OutDataTypeStr=Inherit: Same as first input
  Sum : Sum  Inputs=|++  SaturateOnIntegerOverflow=on
  Transpose : Math  Operator=transpose  SaturateOnIntegerOverflow=on
  Vbxw : aerolibutil/3x3 Cross Product  SystemSampleTime=-1
  Velocity Conversion : aerolibconvert2/Velocity Conversion  SystemSampleTime=-1  IU=m/s  OU=m/s
  Velocity Conversion1 : aerolibconvert2/Velocity Conversion  SystemSampleTime=-1  IU=m/s  OU=m/s
  m_dot : Ground
  mass : Ground
  "p,q,r " : Integrator  InitialCondition=pm_0
  "transform to Inertial axes " : Subsystem
      mask Type: Vector Transformation
      mask Display: disp('L_EB')
  ub,vb,wb : Integrator  InitialCondition=convvel(Vm_0,'m/s','m/s')
  xe,ye,ze : Integrator  InitialCondition=xme_0
  Ve : Outport
  Xe : Outport  Port=2
  Euler : Outport  Port=3
  DCM : Outport  Port=4
  Vb : Outport  Port=5
  p,q,r : Outport  Port=6
  pdot,qdot,rdot : Outport  Port=7
  Ab : Outport  Port=8
  wires:
  Velocity Conversion1/1 -> Ve/1
  Velocity Conversion/1 -> Vb/1
  "Determine Force,  Mass & Inertia"/3 -> Calculate omega_dot/2
  Calculate DCM & Euler Angles/2 -> Euler/1
  Vbxw/1 -> Sum/2
  ub,vb,wb/1 -> Velocity Conversion/1, "transform to Inertial axes "/1(x y z), Vbxw/1, "Determine Force,  Mass & Inertia"/1
  Sum/1 -> ub,vb,wb/1
  xe,ye,ze/1 -> Xe/1
  "transform to Inertial axes "/1(Ve) -> Velocity Conversion1/1, xe,ye,ze/1
  "p,q,r "/1 -> Vbxw/2, p,q,r/1, Calculate DCM & Euler Angles/1, Calculate omega_dot/1
  Moments/1 -> Calculate omega_dot/3
  Forces/1 -> "Determine Force,  Mass & Inertia"/2
  Product/1 -> Sum/1, Ab/1
  Calculate DCM & Euler Angles/1 -> DCM/1, Transpose/1
  Transpose/1 -> "transform to Inertial axes "/2(transform coefficients)
  mass/1 -> "Determine Force,  Mass & Inertia"/3
  "Determine Force,  Mass & Inertia"/2 -> Product/2
  m_dot/1 -> "Determine Force,  Mass & Inertia"/4
  "Determine Force,  Mass & Inertia"/4 -> Out9/1
  Calculate omega_dot/1 -> pdot,qdot,rdot/1, "p,q,r "/1
  I/1 -> "Determine Force,  Mass & Inertia"/5
  I_dot/1 -> "Determine Force,  Mass & Inertia"/6
  "Determine Force,  Mass & Inertia"/1 -> Product/1

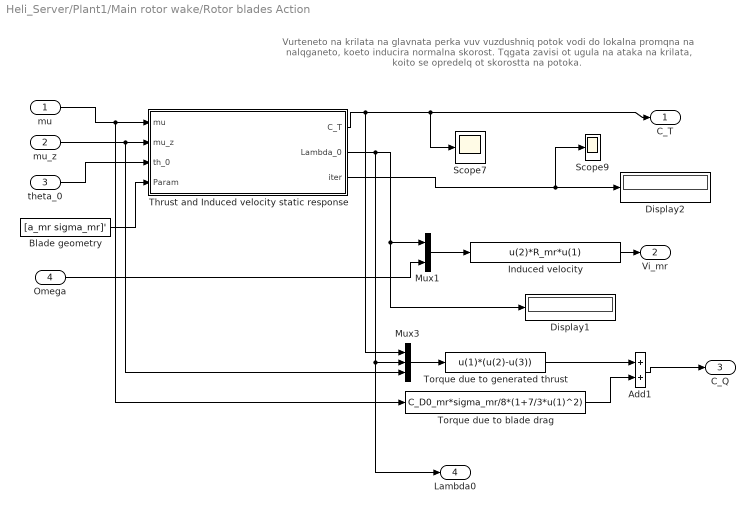
== system Heli_Server/Plant1/Main rotor wake/Rotor blades Action ==
  note: Vurteneto na krilata na glavnata perka vuv vuzdushniq potok
      | vodi do lokalna promqna na nalqganeto, koeto inducira
      | normalna skorost. Tqgata zavisi ot ugula na ataka na krilata, koito
      | se opredelq ot skorostta na potoka.
  mu : Inport
  mu_z : Inport  Port=2
  theta_0 : Inport  Port=3
  Omega : Inport  Port=4
  Add1 : Sum
  Blade geometry : Constant  Value=[a_mr sigma_mr]'
  Display1 : Display
  Display2 : Display
  Induced velocity : Fcn  Expr=u(2)*R_mr*u(1)
  Mux1 : Mux  Inputs=2
  Mux3 : Mux  Inputs=3
  Scope7 : Scope
      settings: TimeRange=10  YMin=0.0015  YMax=0.0055  SaveName=ScopeData20
  Scope9 : Scope
      settings: SaveName=ScopeData22
  Thrust and Induced velocity static response : Stateflow chart  TreatAsAtomicUnit=on
  Torque due to blade drag : Fcn  Expr=C_D0_mr*sigma_mr/8*(1+7/3*u(1)^2)
  Torque due to generated thrust : Fcn  Expr=u(1)*(u(2)-u(3))
  C_T : Outport
  Vi_mr : Outport  Port=2
  C_Q : Outport  Port=3
  Lambda0 : Outport  Port=4
  wires:
  Omega/1 -> Mux1/2
  Mux1/1 -> Induced velocity/1
  Add1/1 -> C_Q/1
  Mux3/1 -> Torque due to generated thrust/1
  Torque due to generated thrust/1 -> Add1/1
  Torque due to blade drag/1 -> Add1/2
  Induced velocity/1 -> Vi_mr/1
  mu_z/1 -> Mux3/3, Thrust and Induced velocity static response/2(mu_z)
  theta_0/1 -> Thrust and Induced velocity static response/3(th_0)
  Blade geometry/1 -> Thrust and Induced velocity static response/4(Param)
  Thrust and Induced velocity static response/1(C_T) -> Mux3/1, Scope7/1, C_T/1
  Thrust and Induced velocity static response/2(Lambda_0) -> Mux1/1, Display1/1, Mux3/2, Lambda0/1
  Thrust and Induced velocity static response/3(iter) -> Display2/1, Scope9/1
  mu/1 -> Torque due to blade drag/1, Thrust and Induced velocity static response/1(mu)

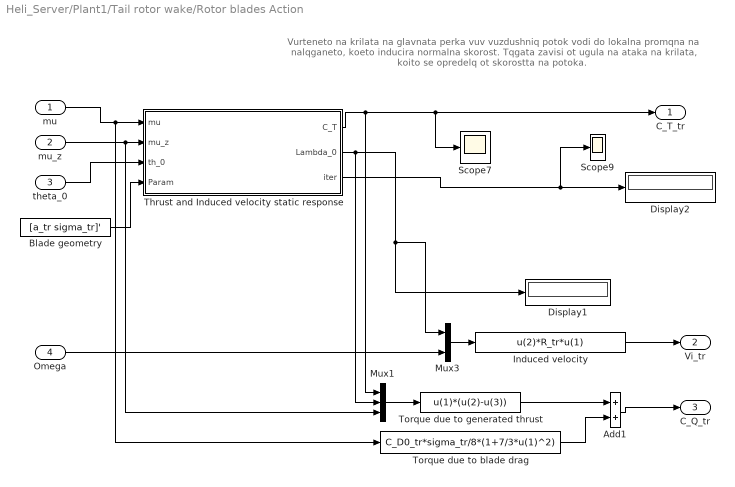
== system Heli_Server/Plant1/Tail rotor wake/Rotor blades Action ==
  note: Vurteneto na krilata na glavnata perka vuv vuzdushniq potok
      | vodi do lokalna promqna na nalqganeto, koeto inducira
      | normalna skorost. Tqgata zavisi ot ugula na ataka na krilata, koito
      | se opredelq ot skorostta na potoka.
  mu : Inport
  mu_z : Inport  Port=2
  theta_0 : Inport  Port=3
  Omega : Inport  Port=4
  Add1 : Sum
  Blade geometry : Constant  Value=[a_tr sigma_tr]'
  Display1 : Display
  Display2 : Display
  Induced velocity : Fcn  Expr=u(2)*R_tr*u(1)
  Mux1 : Mux  Inputs=3
  Mux3 : Mux  Inputs=2
  Scope7 : Scope
      settings: TimeRange=10  YMin=0.0015  YMax=0.0055  SaveName=ScopeData20
  Scope9 : Scope
      settings: SaveName=ScopeData22
  Thrust and Induced velocity static response : Stateflow chart  TreatAsAtomicUnit=on
  Torque due to blade drag : Fcn  Expr=C_D0_tr*sigma_tr/8*(1+7/3*u(1)^2)
  Torque due to generated thrust : Fcn  Expr=u(1)*(u(2)-u(3))
  C_T_tr : Outport
  Vi_tr : Outport  Port=2
  C_Q_tr : Outport  Port=3
  wires:
  mu/1 -> Thrust and Induced velocity static response/1(mu), Torque due to blade drag/1
  Thrust and Induced velocity static response/3(iter) -> Scope9/1, Display2/1
  Thrust and Induced velocity static response/2(Lambda_0) -> Display1/1, Mux3/1, Mux1/2
  Thrust and Induced velocity static response/1(C_T) -> C_T_tr/1, Scope7/1, Mux1/1
  Blade geometry/1 -> Thrust and Induced velocity static response/4(Param)
  theta_0/1 -> Thrust and Induced velocity static response/3(th_0)
  mu_z/1 -> Thrust and Induced velocity static response/2(mu_z), Mux1/3
  Induced velocity/1 -> Vi_tr/1
  Mux3/1 -> Induced velocity/1
  Omega/1 -> Mux3/2
  Torque due to blade drag/1 -> Add1/2
  Torque due to generated thrust/1 -> Add1/1
  Mux1/1 -> Torque due to generated thrust/1
  Add1/1 -> C_Q_tr/1

== system Heli_Server/Plant1/Fuselage/6DoF (Euler Angles)/transform to Inertial axes  ==
  x y z : Inport
  transform coefficients : Inport  Port=2
  Product : Product  Multiplication=Matrix(*)  SaturateOnIntegerOverflow=on  InputSameDT=on  OutDataTypeStr=Inherit: Same as first input
  Reshape1 : Reshape  OutputDimensionality=Column vector (2-D)
  Reshape2 : Reshape
  Ve : Outport
  wires:
  Product/1 -> Reshape2/1
  transform coefficients/1 -> Product/1
  x y z/1 -> Reshape1/1
  Reshape1/1 -> Product/2
  Reshape2/1 -> Ve/1

== matlab function Plant1/Tail rotor wake/Rotor blades Action/Thrust and Induced velocity static response ==
  data: mu input double; mu_z input double; C_T output double; th_0 input double; Lambda_0 output double; Param input double; iter output double
function [C_T,Lambda_0,iter]  = Calc_Blade_Action(mu, mu_z, th_0, Param)
%#eml

a=Param(1);
sigma=Param(2);

e_L0=10;
eta_w=0.9;
L0_old=0;
L0_new=0.01;
CT_old=0;
CT_max=0.05;
iter=0;

while (e_L0>1e-14)
    L0_old=L0_new;
    LAM=sqrt(mu^2+(L0_old-mu_z)^2);
    h_old=-LAM*(24*eta_w*L0_old*LAM+a*sigma*(-2*th_0+3*L0_old+3*th_0*mu^2-3*mu_z))/(3*(8*eta_w*(LAM^2+L0_old*(L0_old-mu_z))+a*LAM*sigma)+1e-6);
    L0_new=L0_old+0.6*h_old;
    e_L0=(L0_new-L0_old)^2;
    iter=iter+1;
    if (iter>500) break; end
end

CT_old=a*sigma/2*(th_0*(1/3+mu^2/2)+(mu_z-L0_old)/2);
if CT_old>CT_max
    CT_old=CT_max;
elseif CT_old<-CT_max
    CT_old=-CT_max;
end

Lambda_0=L0_old;
C_T=CT_old;

== matlab function Plant1/Main rotor wake/Main rotor flow affects tail rotor flow ==
  data: Air_velocity input double; Vi_mr input double; tr_flow output double; Geom_Param input double; K_lambda output double
function [tr_flow,K_lambda]  = fcn(Air_velocity, Vi_mr, Geom_Param)
%#eml

%calculate the vertical direction of main rotor flow
Flow_mr_dir=Air_velocity(1)/(Vi_mr-Air_velocity(3));
g_i=Geom_Param(1);
g_f=Geom_Param(2);
K_lambda = 0;
if (Vi_mr<Air_velocity(3)) || (Flow_mr_dir <= g_i)
    K_lambda = 0;
elseif (Flow_mr_dir > g_i) && (Flow_mr_dir < g_f)
    K_lambda = 1.5*(Flow_mr_dir - g_i)/(g_f - g_i);
elseif (Flow_mr_dir >= g_f)
    K_lambda = 1.5;
end

tr_flow=K_lambda*Vi_mr;

== matlab function Plant1/Main rotor wake/Rotor blades Action/Thrust and Induced velocity static response ==
  data: mu input double; mu_z input double; C_T output double; th_0 input double; Lambda_0 output double; Param input double; iter output double
function [C_T,Lambda_0,iter]  = Calc_Blade_Action(mu, mu_z, th_0, Param)
%#eml

a=Param(1);
sigma=Param(2);

e_L0=10;
eta_w=0.9;
L0_old=0;
L0_new=0.01;
CT_old=0;
CT_max=0.0055;
iter=0;

while (e_L0>1e-14)
    L0_old=L0_new;
    LAM=sqrt(mu^2+(L0_old-mu_z)^2);
    h_old=-LAM*(24*eta_w*L0_old*LAM+a*sigma*(-2*th_0+3*L0_old+3*th_0*mu^2-3*mu_z))/(3*(8*eta_w*(LAM^2+L0_old*(L0_old-mu_z))+a*LAM*sigma)+1e-6);
    L0_new=L0_old+0.6*h_old;
    e_L0=(L0_new-L0_old)^2;
    iter=iter+1;
    if (iter>500) break; end
end

CT_old=a*sigma/2*(th_0*(1/3+mu^2/2)+(mu_z-L0_old)/2);
if CT_old>CT_max
    CT_old=CT_max;
elseif CT_old<-CT_max
    CT_old=-CT_max;
end

Lambda_0=L0_old;
C_T=CT_old;
